simulink model "PMSM"  (R2019b)
settings: Solver=VariableStepAuto  StartTime=0.0  StopTime=2  RelTol=1e-3
InitFcn:
  | P = 8
  | flux = 0.2068
  | 
  | Vd = 600
  | 
  | Rs = 1.477
  | R=1.477
  | Lq = 0.0225
  | Ld = 0.01975
  | 
  | 
  | B=0.0034
  | J=0.0015806
  | 
  | PM  = 75;
  | Wc = 3920;
  | 
  | PI_q = tand(PM - 90 + atand((Wc*Lq)/R));
  | Ki_q = (Wc * sqrt(((R)^2)+((Wc*Lq)^2))/sqrt(1+(PI_q)^2));
  | Kp_q = (PI_q * Ki_q)/Wc;
  | PI_d = tand(PM - 90 + atand((Wc*Ld)/R));
  | Ki_d = (Wc * sqrt(((R)^2)+((Wc*Ld)^2))/sqrt(1+(PI_d)^2));
  | Kp_d = (PI_d * Ki_d)/Wc;
  | 
  | 
  | Wc=2*pi*42;
  | PM=78;
  | wpi=tand(PM-90+atand((Wc*180/pi)*J/B));
  | Ki= (Wc * sqrt(B^2 + (Wc*J)^2))/(sqrt(1+(wpi)^2));
  | Kp= (wpi*Ki)/(Wc);
libraries: powerlib_meascontrol x5
settings Model: Creator=kanth  LastModifiedBy=kanth

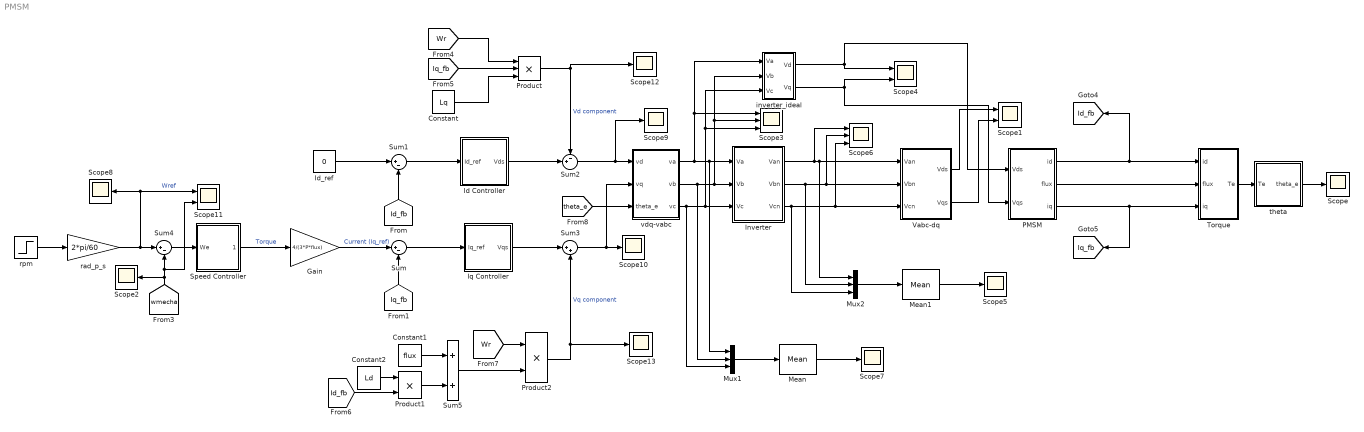
== system PMSM ==
  Constant : Constant  Value=Lq
  Constant1 : Constant  Value=flux
  Constant2 : Constant  Value=Ld
  Gain : Gain  Gain=4/(3*P*flux)
  Id Controller : Subsystem
  Id_ref : Constant  Value=0
  Inverter : Subsystem
  Iq Controller : Subsystem
  Mean : powerlib_meascontrol/Measurements/Mean  Freq=5000  Vinit=0  Ts=0
      settings: SourceProductName=Simscape Electrical
  Mean1 : powerlib_meascontrol/Measurements/Mean  Freq=5000  Vinit=0  Ts=0
      settings: SourceProductName=Simscape Electrical
  Mux1 : Mux  Inputs=3
  Mux2 : Mux  Inputs=3
  PMSM : Subsystem
  Product : Product  Inputs=3
  Product1 : Product
  Product2 : Product
  Scope{,2,5,7..10,12..13} (9 alike) : Scope
  Scope1 : Scope  NumInputPorts=2
  Scope11 : Scope  NumInputPorts=2
  Scope3 : Scope  NumInputPorts=3
  Scope4 : Scope  NumInputPorts=2
  Scope6 : Scope  NumInputPorts=3
  Speed Controller : Subsystem
  Sum : Sum  Inputs=|+-
  Sum1 : Sum  Inputs=|+-
  Sum2 : Sum  Inputs=-+|
  Sum3 : Sum  Inputs=|++
  Sum4 : Sum  Inputs=|+-
  Sum5 : Sum
  Torque : Subsystem
  Vabc-dq : Subsystem
  inverter_ideal : Subsystem
  rad_p_s : Gain  Gain=2*pi/60
  rpm : Step  Time=1.5  Before=1000  After=-1000  SampleTime=0
  theta : Subsystem
  vdq-vabc : Subsystem
  tag scope: Id_fb=global, Iq_fb=global
  wires:
  Sum/1 -> Iq Controller/1(Iq_ref)
  Sum1/1 -> Id Controller/1(Id_ref)
  Iq Controller/1(Vqs) -> Sum3/1
  Sum2/1 -> Scope9/1, vdq-vabc/1(vd)
  Sum3/1 -> Scope10/1, vdq-vabc/2(vq)
  [Id_fb] -> Sum1/2
  [Iq_fb] -> Sum/2
  Id_ref/1 -> Sum1/1
  rad_p_s/1 -> Scope11/1, Scope8/1, Sum4/1  "Wref"
  [wmecha] -> Scope11/2, Sum4/2, Scope2/1
  [Iq_fb] -> Product/2
  [Wr] -> Product/1
  Constant/1 -> Product/3
  Product/1 -> Scope12/1, Sum2/1  "Vd component"
  Id Controller/1(Vds) -> Sum2/2
  Constant1/1 -> Sum5/1
  Constant2/1 -> Product1/1
  [Id_fb] -> Product1/2
  Product1/1 -> Sum5/2
  Sum5/1 -> Product2/2
  [Wr] -> Product2/1
  [theta_e] -> vdq-vabc/3(theta_e)
  Product2/1 -> Scope13/1, Sum3/2  "Vq component"
  rpm/1 -> rad_p_s/1
  Inverter/1(Van) -> Scope6/1, Mux2/1, Vabc-dq/1(Van)
  Inverter/2(Vbn) -> Mux2/2, Scope6/2, Vabc-dq/2(Vbn)
  Inverter/3(Vcn) -> Mux2/3, Scope6/3, Vabc-dq/3(Vcn)
  PMSM/1(id) -> Torque/1(id), [Id_fb]
  PMSM/3(iq) -> [Iq_fb], Torque/3(iq)
  PMSM/2(flux) -> Torque/2(flux)
  Torque/1(Te) -> theta/1(Te)
  theta/1(theta_e) -> Scope/1
  Speed Controller/1(Torque) -> Gain/1  "Torque"
  inverter_ideal/1(Vd) -> PMSM/1(Vds), Scope4/1
  inverter_ideal/2(Vq) -> PMSM/2(Vqs), Scope4/2
  Mean/1 -> Scope7/1
  Mux1/1 -> Mean/1
  vdq-vabc/3(vc) -> Mux1/3, Scope3/3, inverter_ideal/3(Vc), Inverter/3(Vc)
  vdq-vabc/2(vb) -> Mux1/2, Scope3/2, inverter_ideal/2(Vb), Inverter/2(Vb)
  vdq-vabc/1(va) -> Mux1/1, Inverter/1(Va), Scope3/1, inverter_ideal/1(Va)
  Mux2/1 -> Mean1/1
  Mean1/1 -> Scope5/1
  Sum4/1 -> Speed Controller/1(We)
  Gain/1 -> Sum/1  "Current (Iq_ref)"
  Vabc-dq/1(Vds) -> Scope1/1
  Vabc-dq/2(Vqs) -> Scope1/2

== system PMSM/Id Controller ==
  Id_ref : Inport
  "  1" : Gain  Gain=Ki_d
  " 1" : Gain  Gain=Kp_d
  Integrator1 : Integrator  LimitOutput=on  UpperSaturationLimit=220  LowerSaturationLimit=-220
  Saturation1 : Saturate  UpperLimit=240  LowerLimit=-240
  Sum5 : Sum  Inputs=|++
  Vds : Outport
  wires:
  "  1"/1 -> Integrator1/1
  Id_ref/1 -> " 1"/1, "  1"/1
  Integrator1/1 -> Sum5/2
  Sum5/1 -> Saturation1/1
  Saturation1/1 -> Vds/1
  " 1"/1 -> Sum5/1

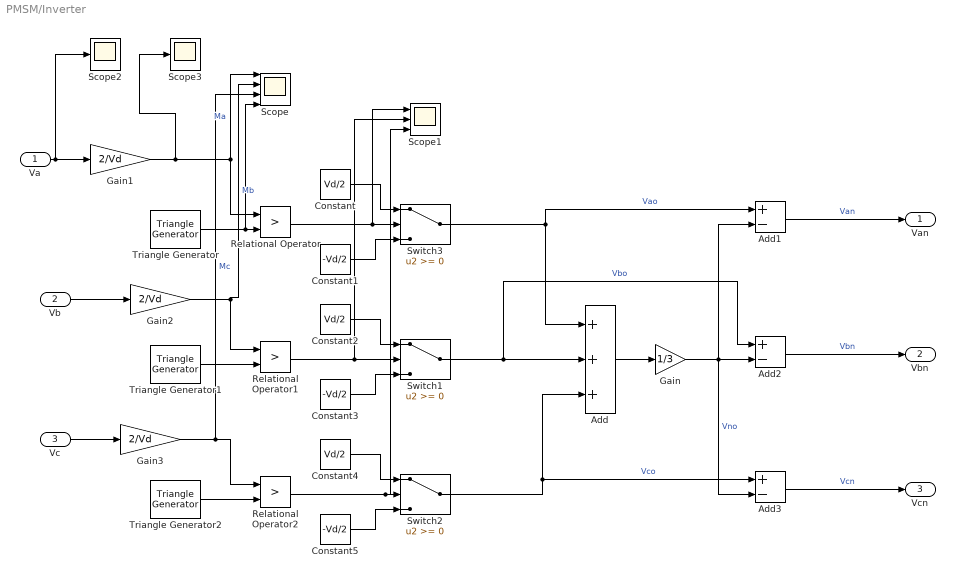
== system PMSM/Inverter ==
  Va : Inport
  Vb : Inport  Port=2
  Vc : Inport  Port=3
  Add : Sum  Inputs=+++
  Add1 : Sum  Inputs=+-
  Add2 : Sum  Inputs=+-
  Add3 : Sum  Inputs=+-
  Constant : Constant  Value=Vd/2
  Constant1 : Constant  Value=-Vd/2
  Constant2 : Constant  Value=Vd/2
  Constant3 : Constant  Value=-Vd/2
  Constant4 : Constant  Value=Vd/2
  Constant5 : Constant  Value=-Vd/2
  Gain : Gain  Gain=1/3
  Gain1 : Gain  Gain=2/Vd
  Gain2 : Gain  Gain=2/Vd
  Gain3 : Gain  Gain=2/Vd
  Relational Operator : RelationalOperator  Operator=>  OutDataTypeStr=boolean  RndMeth=Simplest
  Relational Operator1 : RelationalOperator  Operator=>  OutDataTypeStr=boolean  RndMeth=Simplest
  Relational Operator2 : RelationalOperator  Operator=>  OutDataTypeStr=boolean  RndMeth=Simplest
  Scope : Scope  NumInputPorts=4
  Scope1 : Scope  NumInputPorts=3
  Scope2 : Scope
  Scope3 : Scope
  Switch1 : Switch
  Switch2 : Switch
  Switch3 : Switch
  Triangle Generator : powerlib_meascontrol/Pulse & Signal Generators/Triangle Generator  Freq=5000  Phase=0  Ts=0
      settings: SourceProductName=Simscape Electrical
  Triangle Generator1 : powerlib_meascontrol/Pulse & Signal Generators/Triangle Generator  Freq=5000  Phase=0  Ts=0
      settings: SourceProductName=Simscape Electrical
  Triangle Generator2 : powerlib_meascontrol/Pulse & Signal Generators/Triangle Generator  Freq=5000  Phase=0  Ts=0
      settings: SourceProductName=Simscape Electrical
  Van : Outport
  Vbn : Outport  Port=2
  Vcn : Outport  Port=3
  wires:
  Relational Operator1/1 -> Scope1/2, Switch1/2
  Switch3/1 -> Add1/1, Add/1  "Vao"
  Switch1/1 -> Add/2, Add2/1  "Vbo"
  Constant2/1 -> Switch1/1
  Constant/1 -> Switch3/1
  Gain/1 -> Add3/2, Add2/2, Add1/2  "Vno"
  Constant3/1 -> Switch1/3
  Switch2/1 -> Add/3, Add3/1  "Vco"
  Relational Operator/1 -> Scope1/1, Switch3/2
  Add3/1 -> Vcn/1  "Vcn"
  Triangle Generator/1 -> Scope/4, Relational Operator/2
  Triangle Generator2/1 -> Relational Operator2/2
  Constant1/1 -> Switch3/3
  Constant5/1 -> Switch2/3
  Constant4/1 -> Switch2/1
  Va/1 -> Scope2/1, Gain1/1
  Add/1 -> Gain/1
  Triangle Generator1/1 -> Relational Operator1/2
  Relational Operator2/1 -> Scope1/3, Switch2/2
  Vc/1 -> Gain3/1
  Add1/1 -> Van/1  "Van"
  Vb/1 -> Gain2/1
  Add2/1 -> Vbn/1  "Vbn"
  Gain1/1 -> Scope3/1, Scope/1, Relational Operator/1  "Ma"
  Gain2/1 -> Scope/2, Relational Operator1/1  "Mb"
  Gain3/1 -> Relational Operator2/1, Scope/3  "Mc"

== system PMSM/Iq Controller ==
  Iq_ref : Inport
  " " : Gain  Gain=Kp_q
  "  " : Gain  Gain=Ki_q
  Integrator : Integrator  LimitOutput=on  UpperSaturationLimit=220  LowerSaturationLimit=-220
  Saturation : Saturate  UpperLimit=240  LowerLimit=-240
  Sum2 : Sum  Inputs=|++
  Vqs : Outport
  wires:
  "  "/1 -> Integrator/1
  Sum2/1 -> Saturation/1
  " "/1 -> Sum2/1
  Integrator/1 -> Sum2/2
  Iq_ref/1 -> "  "/1, " "/1
  Saturation/1 -> Vqs/1  "Voltage"

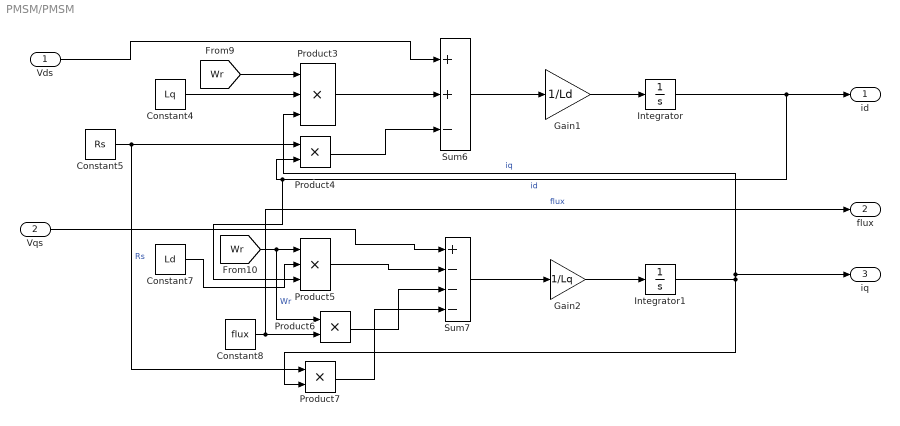
== system PMSM/PMSM ==
  Vds : Inport
  Vqs : Inport  Port=2
  Constant4 : Constant  Value=Lq
  Constant5 : Constant  Value=Rs
  Constant7 : Constant  Value=Ld
  Constant8 : Constant  Value=flux
  Gain1 : Gain  Gain=1/Ld
  Gain2 : Gain  Gain=1/Lq
  Integrator : Integrator
  Integrator1 : Integrator
  Product3 : Product  Inputs=3
  Product4 : Product
  Product5 : Product  Inputs=3
  Product6 : Product
  Product7 : Product
  Sum6 : Sum  Inputs=++-
  Sum7 : Sum  Inputs=+---
  id : Outport
  flux : Outport  Port=2
  iq : Outport  Port=3
  wires:
  Sum7/1 -> Gain2/1
  [Wr] -> Product6/1, Product5/1  "Wr"
  Product3/1 -> Sum6/2
  Constant8/1 -> flux/1, Product6/2  "flux"
  Gain1/1 -> Integrator/1
  Product4/1 -> Sum6/3
  Constant7/1 -> Product5/2
  Gain2/1 -> Integrator1/1
  Constant5/1 -> Product7/1, Product4/1  "Rs"
  Product6/1 -> Sum7/3
  Constant4/1 -> Product3/2
  Vqs/1 -> Sum7/1
  [Wr] -> Product3/1
  Sum6/1 -> Gain1/1
  Product7/1 -> Sum7/4
  Product5/1 -> Sum7/2
  Integrator/1 -> Product5/3, Product4/2, id/1  "id"
  Integrator1/1 -> Product3/3, iq/1, Product7/2  "iq"
  Vds/1 -> Sum6/1

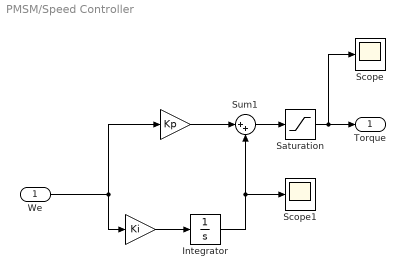
== system PMSM/Speed Controller ==
  We : Inport
  " " : Gain  Gain=Kp
  "  " : Gain  Gain=Ki
  Integrator : Integrator  LimitOutput=on  UpperSaturationLimit=10  LowerSaturationLimit=-10
  Saturation : Saturate  UpperLimit=12  LowerLimit=-12
  Scope : Scope
  Scope1 : Scope
  Sum1 : Sum  Inputs=|++
  Torque : Outport
  wires:
  Saturation/1 -> Scope/1, Torque/1
  "  "/1 -> Integrator/1
  Integrator/1 -> Sum1/2, Scope1/1
  We/1 -> "  "/1, " "/1
  " "/1 -> Sum1/1
  Sum1/1 -> Saturation/1

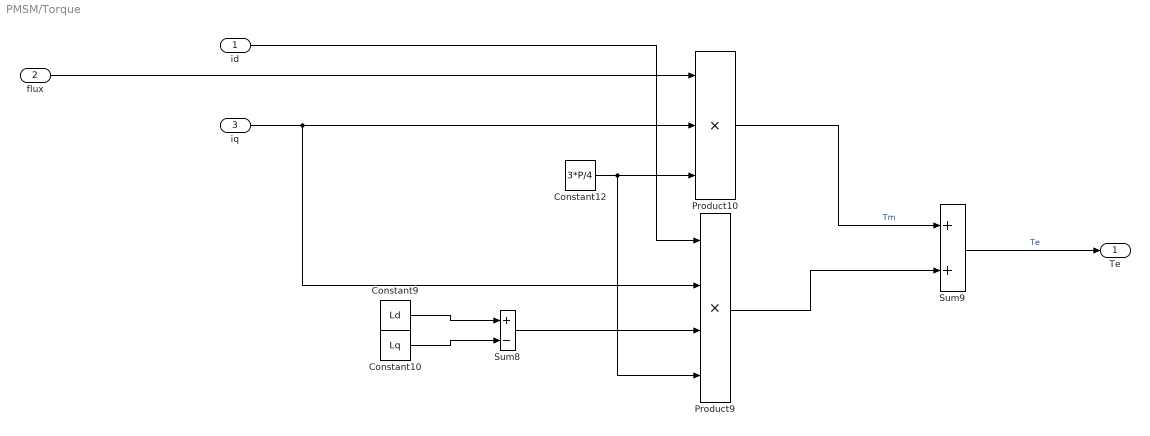
== system PMSM/Torque ==
  id : Inport
  flux : Inport  Port=2
  iq : Inport  Port=3
  Constant10 : Constant  Value=Lq
  Constant12 : Constant  Value=3*P/4
  Constant9 : Constant  Value=Ld
  Product10 : Product  Inputs=3
  Product9 : Product  Inputs=4
  Sum8 : Sum  Inputs=+-
  Sum9 : Sum
  Te : Outport
  wires:
  id/1 -> Product9/1
  iq/1 -> Product9/2, Product10/2
  flux/1 -> Product10/1
  Constant12/1 -> Product9/4, Product10/3
  Product9/1 -> Sum9/2
  Sum8/1 -> Product9/3
  Constant10/1 -> Sum8/2
  Product10/1 -> Sum9/1  "Tm"
  Constant9/1 -> Sum8/1
  Sum9/1 -> Te/1  "Te"

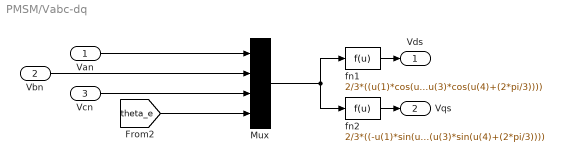
== system PMSM/Vabc-dq ==
  Van : Inport
  Vbn : Inport  Port=2
  Vcn : Inport  Port=3
  Mux : Mux
  fn1 : Fcn  Expr=2/3*((u(1)*cos(u(4)))+(u(2)*cos(u(4)-(2*pi/3)))+(u(3)*cos(u(4)+(2*pi/3))))
  fn2 : Fcn  Expr=2/3*((-u(1)*sin(u(4)))-(u(2)*sin(u(4)-(2*pi/3)))-(u(3)*sin(u(4)+(2*pi/3))))
  Vds : Outport
  Vqs : Outport  Port=2
  wires:
  Vcn/1 -> Mux/3
  Van/1 -> Mux/1
  [theta_e] -> Mux/4
  fn1/1 -> Vds/1
  Mux/1 -> fn1/1, fn2/1
  Vbn/1 -> Mux/2
  fn2/1 -> Vqs/1

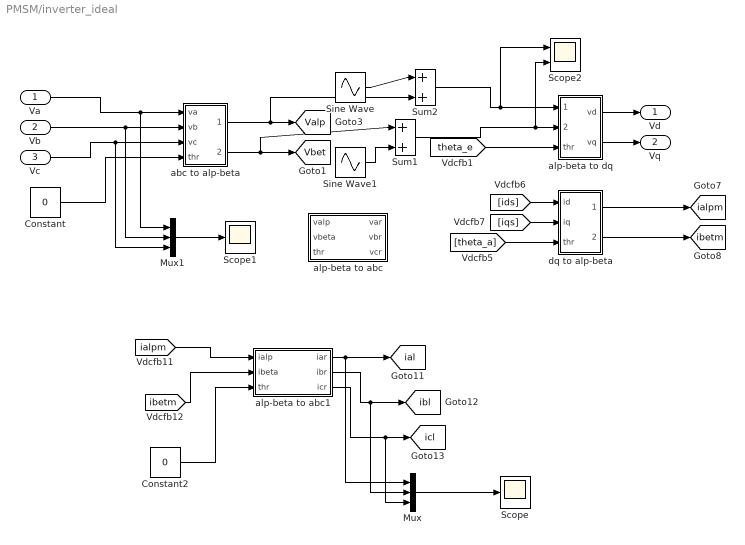
== system PMSM/inverter_ideal ==
  Va : Inport
  Vb : Inport  Port=2
  Vc : Inport  Port=3
  Constant : Constant  Value=0
  Constant2 : Constant  Value=0
  Mux : Mux  Inputs=3
  Mux1 : Mux  Inputs=3
  Scope : Scope
  Scope1 : Scope
  Scope2 : Scope  NumInputPorts=2
  Sine Wave : Sin  Amplitude=0  Frequency=2*pi*1000  SampleTime=0
  Sine Wave1 : Sin  Amplitude=0  Frequency=2*pi*1000  Phase=pi/2  SampleTime=0
  Sum1 : Sum  Inputs=|++
  Sum2 : Sum  Inputs=|++
  abc to alp-beta : Subsystem
  alp-beta to abc : Subsystem
  alp-beta to abc1 : Subsystem
  alp-beta to dq : Subsystem
  dq to alp-beta : Subsystem
  Vd : Outport
  Vq : Outport  Port=2
  tag scope: Valp=global, Vbet=global, ial=global, ialpm=global, ibetm=global, ibl=global, icl=global
  wires:
  abc to alp-beta/2(vbeta) -> [Vbet], Sum1/1
  abc to alp-beta/1(valp) -> [Valp], Sum2/2
  Constant/1 -> abc to alp-beta/4(thr)
  Vb/1 -> abc to alp-beta/2(vb), Mux1/2
  Va/1 -> abc to alp-beta/1(va), Mux1/1
  Vc/1 -> abc to alp-beta/3(vc), Mux1/3
  [theta_e] -> alp-beta to dq/3(thr)
  [theta_a] -> dq to alp-beta/3(thr)
  alp-beta to dq/1(vd) -> Vd/1
  alp-beta to dq/2(vq) -> Vq/1
  [ids] -> dq to alp-beta/1(id)
  [iqs] -> dq to alp-beta/2(iq)
  dq to alp-beta/1(ialp) -> [ialpm]
  dq to alp-beta/2(ibet) -> [ibetm]
  Sine Wave/1 -> Sum2/1
  Sum2/1 -> Scope2/1, alp-beta to dq/1(valp)
  Sine Wave1/1 -> Sum1/2
  Sum1/1 -> Scope2/2, alp-beta to dq/2(vbet)
  [ialpm] -> alp-beta to abc1/1(ialp)
  [ibetm] -> alp-beta to abc1/2(ibeta)
  Constant2/1 -> alp-beta to abc1/3(thr)
  alp-beta to abc1/1(iar) -> [ial], Mux/1
  alp-beta to abc1/2(ibr) -> [ibl], Mux/2
  alp-beta to abc1/3(icr) -> [icl], Mux/3
  Mux/1 -> Scope/1
  Mux1/1 -> Scope1/1

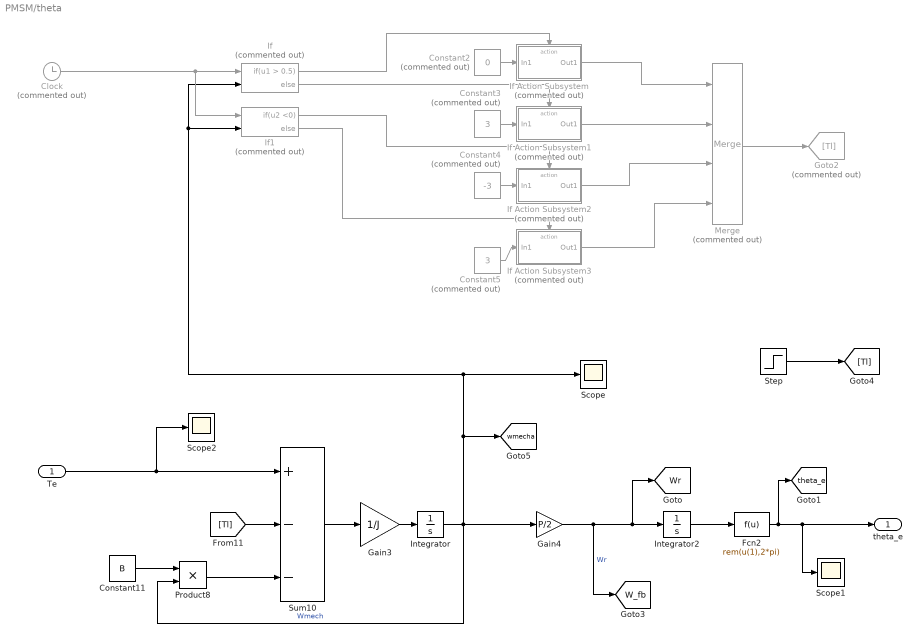
== system PMSM/theta ==
  Te : Inport
  Clock : Clock  Commented=on
  Constant11 : Constant  Value=B
  Constant2 : Constant  Commented=on  Value=0
  Constant3 : Constant  Commented=on  Value=3
  Constant4 : Constant  Commented=on  Value=-3
  Constant5 : Constant  Commented=on  Value=3
  Fcn2 : Fcn  Expr=rem(u(1),2*pi)
  Gain3 : Gain  Gain=1/J
  Gain4 : Gain  Gain=P/2
  Goto2 : Goto  Commented=on  GotoTag=Tl
  If : If  Commented=on  NumInputs=2  IfExpression=u1 > 0.5
  If Action Subsystem : Subsystem  Commented=on  TreatAsAtomicUnit=on
  If Action Subsystem1 : Subsystem  Commented=on  TreatAsAtomicUnit=on
  If Action Subsystem2 : Subsystem  Commented=on  TreatAsAtomicUnit=on
  If Action Subsystem3 : Subsystem  Commented=on  TreatAsAtomicUnit=on
  If1 : If  Commented=on  NumInputs=2  IfExpression=u2 <0
  Integrator : Integrator
  Integrator2 : Integrator
  Merge : Merge  Commented=on  Inputs=4
  Product8 : Product
  Scope : Scope
  Scope1 : Scope
  Scope2 : Scope
  Step : Step  Time=0.5  Before=3  After=10  SampleTime=0
  Sum10 : Sum  Inputs=+--
  theta_e : Outport
  tag scope: W_fb=global, Wr=global, theta_e=global, wmecha=global
  wires:
  Sum10/1 -> Gain3/1
  Gain3/1 -> Integrator/1
  Product8/1 -> Sum10/3
  Integrator2/1 -> Fcn2/1
  Fcn2/1 -> [theta_e], Scope1/1, theta_e/1
  Constant11/1 -> Product8/1
  Gain4/1 -> [W_fb], Integrator2/1, [Wr]  "Wr"
  [Tl] -> Sum10/2
  Te/1 -> Scope2/1, Sum10/1
  Integrator/1 -> [wmecha], Scope/1, If/2, If1/2, Gain4/1, Product8/2  "Wmech"
  If/1 -> If Action Subsystem/Action
  Constant2/1 -> If Action Subsystem/1(In1)
  If Action Subsystem2/1(Out1) -> Merge/3
  Constant4/1 -> If Action Subsystem2/1(In1)
  If Action Subsystem/1(Out1) -> Merge/1
  If Action Subsystem1/1(Out1) -> Merge/2
  If1/1 -> If Action Subsystem2/Action
  Constant5/1 -> If Action Subsystem3/1(In1)
  If1/2 -> If Action Subsystem3/Action
  If/2 -> If Action Subsystem1/Action
  Constant3/1 -> If Action Subsystem1/1(In1)
  Clock/1 -> If1/1, If/1
  If Action Subsystem3/1(Out1) -> Merge/4
  Merge/1 -> Goto2/1
  Step/1 -> [Tl]

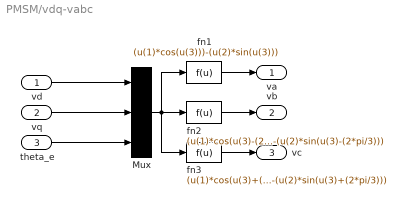
== system PMSM/vdq-vabc ==
  vd : Inport
  vq : Inport  Port=2
  theta_e : Inport  Port=3
  Mux : Mux  Inputs=3
  fn1 : Fcn  Expr=(u(1)*cos(u(3)))-(u(2)*sin(u(3)))
  fn2 : Fcn  Expr=(u(1)*cos(u(3)-(2*pi/3)))-(u(2)*sin(u(3)-(2*pi/3)))
  fn3 : Fcn  Expr=(u(1)*cos(u(3)+(2*pi/3)))-(u(2)*sin(u(3)+(2*pi/3)))
  va : Outport
  vb : Outport  Port=2
  vc : Outport  Port=3
  wires:
  Mux/1 -> fn1/1, fn3/1, fn2/1
  theta_e/1 -> Mux/3
  vq/1 -> Mux/2
  vd/1 -> Mux/1
  fn3/1 -> vc/1
  fn2/1 -> vb/1
  fn1/1 -> va/1

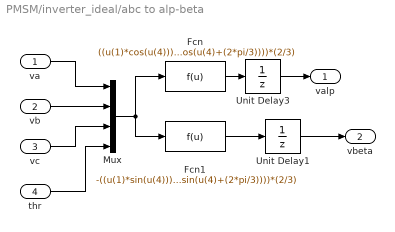
== system PMSM/inverter_ideal/abc to alp-beta ==
  va : Inport
  vb : Inport  Port=2
  vc : Inport  Port=3
  thr : Inport  Port=4
  Fcn : Fcn  Expr=((u(1)*cos(u(4)))+(u(2)*cos(u(4)-2*pi/3))+(u(3)*cos(u(4)+(2*pi/3))))*(2/3)
  Fcn1 : Fcn  Expr=-((u(1)*sin(u(4)))+(u(2)*sin(u(4)-(2*pi/3)))+(u(3)*sin(u(4)+(2*pi/3))))*(2/3)
  Mux : Mux
  Unit Delay1 : UnitDelay  SampleTime=-1
  Unit Delay3 : UnitDelay  SampleTime=-1
  valp : Outport
  vbeta : Outport  Port=2
  wires:
  Fcn1/1 -> Unit Delay1/1
  Fcn/1 -> Unit Delay3/1
  Mux/1 -> Fcn1/1, Fcn/1
  va/1 -> Mux/1
  thr/1 -> Mux/4
  vc/1 -> Mux/3
  vb/1 -> Mux/2
  Unit Delay3/1 -> valp/1
  Unit Delay1/1 -> vbeta/1

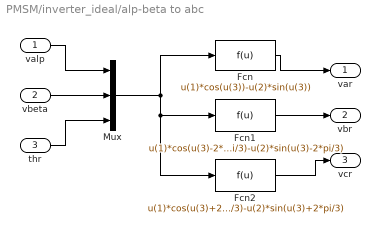
== system PMSM/inverter_ideal/alp-beta to abc ==
  valp : Inport
  vbeta : Inport  Port=2
  thr : Inport  Port=3
  Fcn : Fcn  Expr=u(1)*cos(u(3))-u(2)*sin(u(3))
  Fcn1 : Fcn  Expr=u(1)*cos(u(3)-2*pi/3)-u(2)*sin(u(3)-2*pi/3)
  Fcn2 : Fcn  Expr=u(1)*cos(u(3)+2*pi/3)-u(2)*sin(u(3)+2*pi/3)
  Mux : Mux  Inputs=3
  var : Outport
  vbr : Outport  Port=2
  vcr : Outport  Port=3
  wires:
  valp/1 -> Mux/1
  vbeta/1 -> Mux/2
  thr/1 -> Mux/3
  Mux/1 -> Fcn/1, Fcn1/1, Fcn2/1
  Fcn/1 -> var/1
  Fcn1/1 -> vbr/1
  Fcn2/1 -> vcr/1

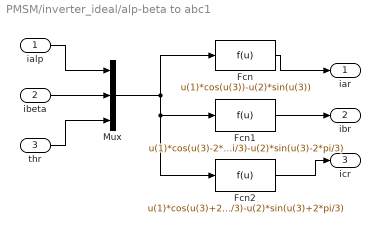
== system PMSM/inverter_ideal/alp-beta to abc1 ==
  ialp : Inport
  ibeta : Inport  Port=2
  thr : Inport  Port=3
  Fcn : Fcn  Expr=u(1)*cos(u(3))-u(2)*sin(u(3))
  Fcn1 : Fcn  Expr=u(1)*cos(u(3)-2*pi/3)-u(2)*sin(u(3)-2*pi/3)
  Fcn2 : Fcn  Expr=u(1)*cos(u(3)+2*pi/3)-u(2)*sin(u(3)+2*pi/3)
  Mux : Mux  Inputs=3
  iar : Outport
  ibr : Outport  Port=2
  icr : Outport  Port=3
  wires:
  Fcn2/1 -> icr/1
  Fcn1/1 -> ibr/1
  Fcn/1 -> iar/1
  Mux/1 -> Fcn2/1, Fcn1/1, Fcn/1
  thr/1 -> Mux/3
  ibeta/1 -> Mux/2
  ialp/1 -> Mux/1

== system PMSM/inverter_ideal/alp-beta to dq ==
  valp : Inport
  vbet : Inport  Port=2
  thr : Inport  Port=3
  Fcn : Fcn  Expr=(u(1)*cos(u(3)))+(u(2)*sin(u(3)))
  Fcn1 : Fcn  Expr=-(u(1)*sin(u(3)))+(u(2)*cos(u(3)))
  Mux : Mux  Inputs=3
  vd : Outport
  vq : Outport  Port=2
  wires:
  vbet/1 -> Mux/2
  thr/1 -> Mux/3
  valp/1 -> Mux/1
  Mux/1 -> Fcn/1, Fcn1/1
  Fcn/1 -> vd/1
  Fcn1/1 -> vq/1

== system PMSM/inverter_ideal/dq to alp-beta ==
  id : Inport
  iq : Inport  Port=2
  thr : Inport  Port=3
  Fcn : Fcn  Expr=(u(1)*cos(u(3)))-(u(2)*sin(u(3)))
  Fcn1 : Fcn  Expr=(u(1)*sin(u(3)))+(u(2)*cos(u(3)))
  Mux : Mux  Inputs=3
  ialp : Outport
  ibet : Outport  Port=2
  wires:
  Fcn1/1 -> ibet/1
  Fcn/1 -> ialp/1
  Mux/1 -> Fcn1/1, Fcn/1
  id/1 -> Mux/1
  thr/1 -> Mux/3
  iq/1 -> Mux/2

== system PMSM/theta/If Action Subsystem ==
  In1 : Inport
  Action Port : ActionPort  ActionPortLabel=if(u1 > 0.5)
  Out1 : Outport
  wires:
  In1/1 -> Out1/1

== system PMSM/theta/If Action Subsystem1 ==
  In1 : Inport
  Action Port : ActionPort  ActionPortLabel=else
  Out1 : Outport
  wires:
  In1/1 -> Out1/1

== system PMSM/theta/If Action Subsystem2 ==
  In1 : Inport
  Action Port : ActionPort  ActionPortLabel=if(u2 <0)
  Out1 : Outport
  wires:
  In1/1 -> Out1/1

== system PMSM/theta/If Action Subsystem3 ==
  In1 : Inport
  Action Port : ActionPort  ActionPortLabel=else
  Out1 : Outport
  wires:
  In1/1 -> Out1/1
